simulink model "D53_LKAS"  (R2018b)
settings: Solver=ode3  StartTime=0.0  StopTime=10.0  FixedStep=0.01  RelTol=1e-3  EnableMultiTasking=on
model workspace (MAT data in the model file):
  MCOS : class17 (value not decoded)
  MCOS : class17 (value not decoded)
  MCOS : class17 (value not decoded)
  MCOS : class17 (value not decoded)
  MCOS : class17 (value not decoded)
  MCOS : class17 (value not decoded)
  MCOS : class17 (value not decoded)
  MCOS : class17 (value not decoded)
  MCOS : class17 (value not decoded)
  MCOS : class17 (value not decoded)
  MCOS : class17 (value not decoded)
  MCOS : class17 (value not decoded)
  MCOS : class17 (value not decoded)
  MCOS : class17 (value not decoded)
  MCOS : class17 (value not decoded)
  MCOS : class17 (value not decoded)
  MCOS : class17 (value not decoded)
  MCOS : class17 (value not decoded)
  MCOS : class17 (value not decoded)
  MCOS : class17 (value not decoded)
  MCOS : class17 (value not decoded)
  MCOS : class17 (value not decoded)
  MCOS : class17 (value not decoded)
  MCOS : class17 (value not decoded)
  MCOS : class17 (value not decoded)
  MCOS : class17 (value not decoded)
  MCOS : class17 (value not decoded)
  MCOS : class17 (value not decoded)
  MCOS : class17 (value not decoded)
  MCOS : class17 (value not decoded)
  MCOS : class17 (value not decoded)
  MCOS : class17 (value not decoded)
  MCOS : class17 (value not decoded)
  MCOS : class17 (value not decoded)
  MCOS : class17 (value not decoded)
  MCOS : class17 (value not decoded)
  MCOS : class17 (value not decoded)
  MCOS : class17 (value not decoded)
  MCOS : class17 (value not decoded)
  MCOS : class17 (value not decoded)
  MCOS : class17 (value not decoded)
  MCOS : class17 (value not decoded)
  MCOS : class17 (value not decoded)
  MCOS : class17 (value not decoded)
  MCOS : class17 (value not decoded)
  MCOS : class17 (value not decoded)
  MCOS : class17 (value not decoded)
  MCOS : class17 (value not decoded)
  MCOS : class17 (value not decoded)
  MCOS : class17 (value not decoded)
  MCOS : class17 (value not decoded)
  MCOS : class17 (value not decoded)
  MCOS : class17 (value not decoded)
  MCOS : class17 (value not decoded)
  MCOS : class17 (value not decoded)
  MCOS : class17 (value not decoded)
  MCOS : class17 (value not decoded)
  MCOS : class17 (value not decoded)
  MCOS : class17 (value not decoded)
  MCOS : class17 (value not decoded)
  MCOS : class17 (value not decoded)
  MCOS : class17 (value not decoded)
  MCOS : class17 (value not decoded)
  MCOS : class17 (value not decoded)
  MCOS : class17 (value not decoded)
  MCOS : class17 (value not decoded)
  MCOS : class17 (value not decoded)
  MCOS : class17 (value not decoded)
  MCOS : class17 (value not decoded)
  MCOS : class17 (value not decoded)
  MCOS : class17 (value not decoded)
  MCOS : class17 (value not decoded)
  MCOS : class17 (value not decoded)
  MCOS : class17 (value not decoded)
  MCOS : class17 (value not decoded)
  MCOS : class17 (value not decoded)
  MCOS : class17 (value not decoded)
  MCOS : class17 (value not decoded)
  MCOS : class17 (value not decoded)
  MCOS : class17 (value not decoded)
  MCOS : class17 (value not decoded)
  MCOS : class17 (value not decoded)
  MCOS : class17 (value not decoded)
  MCOS : class17 (value not decoded)
  MCOS : class17 (value not decoded)
  MCOS : class17 (value not decoded)
  MCOS : class17 (value not decoded)
  MCOS : class17 (value not decoded)
  MCOS : class17 (value not decoded)
values from neighbouring files (symbols this model uses):
  C = who    [Data_Made_Data.m]    (also in Data_Make_Data.m; Data_Process.m)
  LKA_SampleTime = Simulink.Parameter    [Model_NoProtect_Script.m]
  Monitor = find_system(strcat(filename,'/CAN Monitor (CANMon)/Monitor'),'SearchDepth',1,'BlockType','From')    [UpdateMon.m]    (also in UpdateMonAuto.m = find_system(strcat(scriptfile,'/CAN Monitor (CANMon)/Monitor; UpdateMonMdb.m; Update_MonAuto.m = find_system(strcat(scriptfile,'/CAN Monitor (CANMon)/Monitor; Update_MonMdb.m)
undefined symbols (not defined in the file or in its folder): LKA_CarWidth, LKA_StrRatio_C, LKA_Veh2CamL_C, LKA_Veh2CamW_C, LKA_WhlBaseL_C, LL_CompSWA_C, LL_CrvtPrvwT_C, LL_DesDvt_C, LL_DvtComp_C, LL_DvtPrvwT_C, LL_DvtSpdDet_vDvtSpdMin_C, LL_HdAgExT_C, LL_HdAgPrvwT_C, LL_LAccMax_C, LL_LAccRMax_C, LL_LDW_EarliestWarnLine_C, LL_LDW_LatestWarnLine_C, LL_LDWS_SUPPRESS_HEADING, LL_LFClb_TFC_DiffCtlBalance, LL_LFClb_TFC_DiffCtrlMaxSWA, LL_LFClb_TFC_DiffCtrlRatio, LL_LFClb_TFC_facmGainLutGain1_C, LL_LFClb_TFC_facmGainLutGain2_C, LL_LFClb_TFC_facmIntegRatio, LL_LFClb_TFC_facmKlat_C, LL_LFClb_TFC_FfCtlRatio_C, LL_LFClb_TFC_phiIntegCtlMaxSWA_C, LL_LFClb_TFC_tiKlatPrvwT_C, LL_LFClb_TFC_vGainLutVehSpdLwr_C, LL_LFClb_TFC_vGainLutVehSpdUpr_C, LL_LKA_EarliestWarnLine_C, LL_LKA_LatestWarnLine_C, LL_LKAExPrcs_ExitC0Dvt, LL_LKAExPrcs_ExitC0Swt, LL_LKAExPrcs_tiExitTime1, LL_LKAExPrcs_tiExitTime2, LL_LKAExPrcs_tiExitTime3, LL_LKAS_OUT_OF_CONTROL_LAT_VEL, LL_LKAS_OUT_OF_CONTROL_TTLC, LL_LKASWASyn_M0, LL_LKASWASyn_M1, LL_LKASWASyn_M2, LL_LKASWASyn_M3K, LL_LKASWASyn_SWAaddMax, LL_LKASWASyn_T2, LL_LKASWASyn_tiTrqSwaRtTime, LL_LKASWASyn_tiTrqSwaTime, LL_LKASWASyn_TrqMax, LL_LKASWASyn_TrqSwaAddSwt, LL_LKASWASyn_TrqSwaRateDiff, LL_LSpdCompT_C, LL_lStpLngth_C, LL_MAX_DELAY_EPSSTAR_TIME, LL_MAX_DRIVER_TORQUE_DISABLE, LL_MAX_DRIVER_TORQUE_ENABLE, LL_MAX_LANE_WIDTH_DISABLE, LL_MAX_LANE_WIDTH_ENABLE, LL_MAX_LAT_ACC_DISABLE, LL_MAX_LAT_ACC_ENABLE, LL_MAX_LDWS_SPEED_DISABLE ... (+29)
libraries: simulink x134, canmsglib x36, dspstat3 x3, simulink_extras x1
(part 6 of 17)

== system D53_LKAS/SignalBusCreator/bsVehMovInfo ==
  Bus Creator9 : BusCreator  Inputs=10
  CAN Recv (CANRx]) : S-Function  FunctionName=CAN_Rec_P  Parameters=uint8(Module-1),uint32(ID),uint8(Frameformat-1),uint8(Newflag),uint8(FIFO),double(sampletime)  SFunctionDeploymentMode=off  EnableBusSupport=off  mask(CAN_receive){Module=CAN_1, ID=973, Frameformat=Standard (11-bit identifier), Newflag=off, FIFO=off, sampletime=0.01}
      mask prompts: Module "CAN Port:"; ID "CAN Frame ID:"; Frameformat "CAN Frame Format:"; FIFO "Overflow flag"
      mask init:
      | maskdisplay = canrecicon(Module,ID,Frameformat,Newflag,FIFO);
      | set_param(gcb, 'MaskDisplay', maskdisplay);
      mask TypeOptions Module: CAN_0 | CAN_1 | CAN_2 | CAN_3
      mask TypeOptions Frameformat: Standard (11-bit identifier) | Extended (29-bit identifier)
      mask Display: color('blue');text(0.98,0.9,'MPC5675K','horizontalAlignment','right');color('black');text(0.5,0.6,'FlexCAN_1 Receive','horizontalAlignment','center');text(0.5,0.35,'Standard ID:973','horizontalAlignment','center');port_label('output',1,'CAN_Msg');
  CAN Recv (CANRx])1 : S-Function  FunctionName=CAN_Rec_P  Parameters=uint8(Module-1),uint32(ID),uint8(Frameformat-1),uint8(Newflag),uint8(FIFO),double(sampletime)  SFunctionDeploymentMode=off  EnableBusSupport=off  mask(CAN_receive){Module=CAN_1, ID=909, Frameformat=Extended (29-bit identifier), Newflag=off, FIFO=off, sampletime=0.01}
      mask prompts: Module "CAN Port:"; ID "CAN Frame ID:"; Frameformat "CAN Frame Format:"; FIFO "Overflow flag"
      mask init:
      | maskdisplay = canrecicon(Module,ID,Frameformat,Newflag,FIFO);
      | set_param(gcb, 'MaskDisplay', maskdisplay);
      mask TypeOptions Module: CAN_0 | CAN_1 | CAN_2 | CAN_3
      mask TypeOptions Frameformat: Standard (11-bit identifier) | Extended (29-bit identifier)
      mask Display: color('blue');text(0.98,0.9,'MPC5675K','horizontalAlignment','right');color('black');text(0.5,0.6,'FlexCAN_1 Receive','horizontalAlignment','center');text(0.5,0.35,'Extended ID:909','horizontalAlignment','center');port_label('output',1,'CAN_Msg');
  CAN Send1 : S-Function  FunctionName=CAN_Send_P  Parameters=uint8(CAN_Port-1),uint8(CAN_Priority-1),uint8(S_overflow_flag),uint8(S_timestamp),double(sampletime)  SFunctionDeploymentMode=off  EnableBusSupport=off  mask{CAN_Port=CAN_0, CAN_Priority=3, S_overflow_flag=off, S_timestamp=off, sampletime=0.01}
      mask prompts: CAN_Port "CAN Port:"; CAN_Priority "Priority:"; S_overflow_flag "Send overflow flag"; S_timestamp "Send time stamp"
      mask init:
      | maskdisplay = cansendicon(CAN_Port,CAN_Priority,S_overflow_flag,S_timestamp);
      | set_param(gcb, 'MaskDisplay', maskdisplay);
      mask TypeOptions CAN_Port: CAN_0 | CAN_1 | CAN_2 | CAN_3
      mask TypeOptions CAN_Priority: 0 | 1 | 2 | 3 | 4 | 5 | 6 | 7
      mask Display: color('blue');text(0.98,0.9,'MPC5675K','horizontalAlignment','right');color('black');text(0.5,0.6,'FlexCAN_0 Send','horizontalAlignment','center');text(0.5,0.35,'Priority:3','horizontalAlignment','center');port_label('input',1,'CAN_Msg');
  CAN Send2 : S-Function  FunctionName=CAN_Send_P  Parameters=uint8(CAN_Port-1),uint8(CAN_Priority-1),uint8(S_overflow_flag),uint8(S_timestamp),double(sampletime)  SFunctionDeploymentMode=off  EnableBusSupport=off  mask{CAN_Port=CAN_0, CAN_Priority=3, S_overflow_flag=off, S_timestamp=off, sampletime=0.01}
      mask prompts: CAN_Port "CAN Port:"; CAN_Priority "Priority:"; S_overflow_flag "Send overflow flag"; S_timestamp "Send time stamp"
      mask init:
      | maskdisplay = cansendicon(CAN_Port,CAN_Priority,S_overflow_flag,S_timestamp);
      | set_param(gcb, 'MaskDisplay', maskdisplay);
      mask TypeOptions CAN_Port: CAN_0 | CAN_1 | CAN_2 | CAN_3
      mask TypeOptions CAN_Priority: 0 | 1 | 2 | 3 | 4 | 5 | 6 | 7
      mask Display: color('blue');text(0.98,0.9,'MPC5675K','horizontalAlignment','right');color('black');text(0.5,0.6,'FlexCAN_0 Send','horizontalAlignment','center');text(0.5,0.35,'Priority:3','horizontalAlignment','center');port_label('input',1,'CAN_Msg');
  CAN Send3 : S-Function  FunctionName=CAN_Send_P  Parameters=uint8(CAN_Port-1),uint8(CAN_Priority-1),uint8(S_overflow_flag),uint8(S_timestamp),double(sampletime)  SFunctionDeploymentMode=off  EnableBusSupport=off  mask{CAN_Port=CAN_0, CAN_Priority=3, S_overflow_flag=off, S_timestamp=off, sampletime=0.01}
      mask prompts: CAN_Port "CAN Port:"; CAN_Priority "Priority:"; S_overflow_flag "Send overflow flag"; S_timestamp "Send time stamp"
      mask init:
      | maskdisplay = cansendicon(CAN_Port,CAN_Priority,S_overflow_flag,S_timestamp);
      | set_param(gcb, 'MaskDisplay', maskdisplay);
      mask TypeOptions CAN_Port: CAN_0 | CAN_1 | CAN_2 | CAN_3
      mask TypeOptions CAN_Priority: 0 | 1 | 2 | 3 | 4 | 5 | 6 | 7
      mask Display: color('blue');text(0.98,0.9,'MPC5675K','horizontalAlignment','right');color('black');text(0.5,0.6,'FlexCAN_0 Send','horizontalAlignment','center');text(0.5,0.35,'Priority:3','horizontalAlignment','center');port_label('input',1,'CAN_Msg');
  CAN Unpack : canmsglib/CAN Unpack  CANdbFile=D:\Work\02_LKA\LKAS\Documents\D53-PSA1CAN.dbc  MsgList=ESC_3CD_PSA1  MsgName=ESC_3CD_PSA1  MsgIDType=Standard (11-bit identifier)  MsgIdentifier=973  MsgLength=8  SignalInfo=Brake_pedal_disabled_UC_Brake$37$1$2$2$1$0$1$0$-Inf$Inf$#Frame_checksum3CD$60$4$2$2$1$0$1$0$-Inf$Inf$#Lateral_acceleration$8$16$2$1$1$0$5.000000e-02$0$-15$15$#TMC_pressure$52$12$2$2$1$0$1.000000e-01$-55$-55$3.544000e+02$#Yaw_speed$24$16$2$1$1$0$1.000000e-01$0$-100$100$#bits_compute_process_counter3CD$56$4$2$2$1$0$1$0$0$15$#  NSignals=6  IDPort=off  TimestampPort=off  ErrorPort=off  RemotePort=off  LengthPort=off  StatusPort=off  StartBits=str2num('[int32(37);int32(60);int32(8);int32(52);int32(24);int32(56)]')  SignalSizes=str2num('[int32(1);int32(4);int32(16);int32(12);int32(16);int32(4)]')  ByteOrders=str2num('[int32(2);int32(2);int32(2);int32(2);int32(2);int32(2)]')  DataTypes=str2num('[int32(2);int32(2);int32(1);int32(2);int32(1);int32(2)]')  MultiplexTypes=str2num('[int32(1);int32(1);int32(1);int32(1);int32(1);int32(1)]')  MultiplexValues=str2num('[double(0);double(0);double(0);double(0);double(0);double(0)]')  Factors=str2num('[double(1);double(1);double(5.000000e-02);double(1.000000e-01);double(1.000000e-01);double(1)]')  Offsets=str2num('[double(0);double(0);double(0);double(-55);double(0);double(0)]')  Minimums=str2num('[double(-Inf);double(-Inf);double(-15);double(-55);double(-100);double(0)]')  Maximums=str2num('[double(Inf);double(Inf);double(15);double(3.544000e+02);double(100);double(15)]')  ApplyMinMax=off
      settings: SourceProductName=Simulink Real-Time  SourceProductBaseCode=XP  DataFormat=CANdb specified signals
  CAN Unpack1 : canmsglib/CAN Unpack  CANdbFile=D:\Work\02_LKA\LKAS\Documents\D53-PSA1CAN.dbc  MsgList=ESC_38D_PSA1  MsgName=ESC_38D_PSA1  MsgIDType=Standard (11-bit identifier)  MsgIdentifier=909  MsgLength=8  SignalInfo=ABR_dynamic_checksum$40$4$2$2$1$0$1$0$-Inf$Inf$#Vehicle_driving_direction$52$2$2$2$1$0$1$0$-Inf$Inf$#Vehicle_speed_of_wheelsensor$8$16$2$2$1$0$1.000000e-02$0$0$6.553400e+02$#Vehiclespeed_unavailability_flag$50$2$2$2$1$0$1$0$-Inf$Inf$#bits_compute_for_UC_brake$44$4$2$2$1$0$1$0$0$15$#  NSignals=5  IDPort=off  TimestampPort=off  ErrorPort=off  RemotePort=off  LengthPort=off  StatusPort=off  StartBits=str2num('[int32(40);int32(52);int32(8);int32(50);int32(44)]')  SignalSizes=str2num('[int32(4);int32(2);int32(16);int32(2);int32(4)]')  ByteOrders=str2num('[int32(2);int32(2);int32(2);int32(2);int32(2)]')  DataTypes=str2num('[int32(2);int32(2);int32(2);int32(2);int32(2)]')  MultiplexTypes=str2num('[int32(1);int32(1);int32(1);int32(1);int32(1)]')  MultiplexValues=str2num('[double(0);double(0);double(0);double(0);double(0)]')  Factors=str2num('[double(1);double(1);double(1.000000e-02);double(1);double(1)]')  Offsets=str2num('[double(0);double(0);double(0);double(0);double(0)]')  Minimums=str2num('[double(-Inf);double(-Inf);double(0);double(-Inf);double(0)]')  Maximums=str2num('[double(Inf);double(Inf);double(6.553400e+02);double(Inf);double(15)]')  ApplyMinMax=off
      settings: SourceProductName=Simulink Real-Time  SourceProductBaseCode=XP  DataFormat=CANdb specified signals
  CAN Unpack4 : canmsglib/CAN Unpack  CANdbFile=D:\Work\02_LKA\LKAS\Documents\D53-PSA1CAN.dbc  MsgList=GW_32D_PSA1  MsgName=GW_32D_PSA1  MsgIDType=Standard (11-bit identifier)  MsgIdentifier=813  MsgLength=8  SignalInfo=ACCEL_LONGI_CALIB$12$12$2$2$1$0$2.000000e-02$-4.096000e+01$-4.096000e+01$4.092000e+01$#Brake_Pedal_Active$16$2$2$2$1$0$1$0$-Inf$Inf$#Braking_effort$9$1$2$2$1$0$1$0$-Inf$Inf$#ESC_ACC_Status$19$2$2$2$1$0$1$0$-Inf$Inf$#ESC_AEB_Status$10$2$2$2$1$0$1$0$-Inf$Inf$#Message_from_ESC_informing$23$1$2$2$1$0$1$0$-Inf$Inf$#UFC_to_ACC_dynamic_frame$56$4$2$2$1$0$1$0$-Inf$Inf$#Vehicle_Hold_Status$29$2$2$2$1$0$1$0$-Inf$Inf$#Vehicle_detected_as_stationary$21$1$2$2$1$0$1$0$-Inf$Inf$#YawRate_Raw$44$12$2$2$1$0$8.000000e-02$-1.638400e+02$-1.638400e+02$1.636800e+02$#bits_compute_counter_for_UCbrake$60$4$2$2$1$0$1$0$0$15$#  NSignals=11  IDPort=off  TimestampPort=off  ErrorPort=off  RemotePort=off  LengthPort=off  StatusPort=off  StartBits=str2num('[int32(12);int32(16);int32(9);int32(19);int32(10);int32(23);int32(56);int32(29);int32(21);int32(44);int32(60)]')  SignalSizes=str2num('[int32(12);int32(2);int32(1);int32(2);int32(2);int32(1);int32(4);int32(2);int32(1);int32(12);int32(4)]')  ByteOrders=str2num('[int32(2);int32(2);int32(2);int32(2);int32(2);int32(2);int32(2);int32(2);int32(2);int32(2);int32(2)]')  DataTypes=str2num('[int32(2);int32(2);int32(2);int32(2);int32(2);int32(2);int32(2);int32(2);int32(2);int32(2);int32(2)]')  MultiplexTypes=str2num('[int32(1);int32(1);int32(1);int32(1);int32(1);int32(1);int32(1);int32(1);int32(1);int32(1);int32(1)]')  MultiplexValues=str2num('[double(0);double(0);double(0);double(0);double(0);double(0);double(0);double(0);double(0);double(0);double(0)]')  Factors=str2num('[double(2.000000e-02);double(1);double(1);double(1);double(1);double(1);double(1);double(1);double(1);double(8.000000e-02);double(1)]')  Offsets=str2num('[double(-4.096000e+01);double(0);double(0);double(0);double(0);double(0);double(0);double(0);double(0);double(-1.638400e+02);double(0)]')  Minimums=str2num('[double(-4.096000e+01);double(-Inf);double(-Inf);double(-Inf);double(-Inf);double(-Inf);double(-Inf);double(-Inf);double(-Inf);double(-1.638400e+02);double(0)]')  Maximums=str2num('[double(4.092000e+01);double(Inf);double(Inf);double(Inf);double(Inf);double(Inf);double(Inf);double(Inf);double(Inf);double(1.636800e+02);double(15)]')  ApplyMinMax=off
      settings: SourceProductName=Simulink Real-Time  SourceProductBaseCode=XP  DataFormat=CANdb specified signals
  CAN_Receive4 : S-Function  FunctionName=CAN_Rec_P  Parameters=uint8(Module-1),uint32(ID),uint8(Frameformat-1),uint8(Newflag),uint8(FIFO),double(sampletime)  SFunctionDeploymentMode=off  EnableBusSupport=off  mask(CAN_receive){Module=CAN_1, ID=813, Frameformat=Standard (11-bit identifier), Newflag=off, FIFO=off, sampletime=0.01}
      mask prompts: Module "CAN Port:"; ID "CAN Frame ID:"; Frameformat "CAN Frame Format:"; FIFO "Overflow flag"
      mask init:
      | maskdisplay = canrecicon(Module,ID,Frameformat,Newflag,FIFO);
      | set_param(gcb, 'MaskDisplay', maskdisplay);
      mask TypeOptions Module: CAN_0 | CAN_1 | CAN_2 | CAN_3
      mask TypeOptions Frameformat: Standard (11-bit identifier) | Extended (29-bit identifier)
      mask Display: color('blue');text(0.98,0.9,'MPC5675K','horizontalAlignment','right');color('black');text(0.5,0.6,'FlexCAN_1 Receive','horizontalAlignment','center');text(0.5,0.35,'Standard ID:813','horizontalAlignment','center');port_label('output',1,'CAN_Msg');
  Data Type Conversion{1..5,11} (6 alike) : DataTypeConversion  OutDataTypeStr=single
  Data Type Conversion53 : DataTypeConversion  OutDataTypeStr=uint8
  Ground : Ground
  Ground1 : Ground
  Ground2 : Ground
  Rate Transition{,1..5,7} (7 alike) : RateTransition  OutPortSampleTime=0.01
  Terminator{,1..14} (15 alike) : Terminator
  bsVehMovInfo : Outport
  wires:
  CAN Unpack4/1 -> Rate Transition/1
  CAN Unpack/3 -> Rate Transition3/1
  CAN Unpack1/4 -> Rate Transition4/1
  Data Type Conversion2/1 -> Bus Creator9/3  "ESC_YawRate"
  Ground1/1 -> Bus Creator9/4  "ESC_YawRate_Valid"
  Rate Transition3/1 -> Data Type Conversion3/1
  CAN Unpack4/6 -> Terminator7/1
  CAN Unpack/1 -> Terminator2/1
  Rate Transition2/1 -> Data Type Conversion2/1
  Rate Transition7/1 -> Data Type Conversion5/1
  CAN Recv (CANRx])/1 -> CAN Send2/1, CAN Unpack/1
  CAN Unpack1/3 -> Rate Transition7/1
  Data Type Conversion4/1 -> Bus Creator9/5  "ESC_UnYawRate"
  Data Type Conversion11/1 -> Bus Creator9/7  "ESC_LonAcc"
  CAN Unpack/4 -> Rate Transition1/1
  Data Type Conversion53/1 -> Bus Creator9/10  "ESC_VehSpd_Valid"
  Data Type Conversion3/1 -> Bus Creator9/1  "ESC_LatAcc"
  Rate Transition4/1 -> Data Type Conversion53/1
  Rate Transition5/1 -> Data Type Conversion4/1
  Ground2/1 -> Bus Creator9/2  "ESC_LatAcc_Valid"
  Rate Transition1/1 -> Data Type Conversion1/1
  CAN Unpack4/10 -> Rate Transition5/1
  Data Type Conversion1/1 -> Bus Creator9/9  "ESC_Brake_Press"
  CAN Unpack/5 -> Rate Transition2/1
  Rate Transition/1 -> Data Type Conversion11/1
  CAN Unpack4/11 -> Terminator11/1
  CAN Unpack/6 -> Terminator1/1
  Data Type Conversion5/1 -> Bus Creator9/6  "ESC_VehSpd"
  CAN Unpack/2 -> Terminator/1
  CAN Unpack4/4 -> Terminator5/1
  CAN_Receive4/1 -> CAN Send1/1, CAN Unpack4/1
  CAN Unpack4/8 -> Terminator9/1
  CAN Unpack4/7 -> Terminator8/1
  CAN Unpack4/5 -> Terminator6/1
  CAN Unpack4/9 -> Terminator10/1
  CAN Unpack4/2 -> Terminator3/1
  CAN Unpack4/3 -> Terminator4/1
  Bus Creator9/1 -> bsVehMovInfo/1  "bsVehMovInfo"
  Ground/1 -> Bus Creator9/8  "ESC_LonAcc_Valid"
  CAN Recv (CANRx])1/1 -> CAN Send3/1, CAN Unpack1/1
  CAN Unpack1/1 -> Terminator12/1
  CAN Unpack1/2 -> Terminator13/1
  CAN Unpack1/5 -> Terminator14/1

== system D53_LKAS/Clb/Calibration1/Subsystem2 ==
  In1 : Inport
  In2 : Inport  Port=2
  In3 : Inport  Port=3
  In4 : Inport  Port=4
  In5 : Inport  Port=5
  In6 : Inport  Port=6
  In7 : Inport  Port=7
  In8 : Inport  Port=8
  In9 : Inport  Port=9
  In10 : Inport  Port=10
  In11 : Inport  Port=11
  If Action Subsystem : Subsystem  TreatAsAtomicUnit=on
  If Action Subsystem1 : Subsystem  TreatAsAtomicUnit=on
  If Action Subsystem2 : Subsystem  TreatAsAtomicUnit=on
  If Action Subsystem3 : Subsystem  TreatAsAtomicUnit=on
  If Action Subsystem4 : Subsystem  TreatAsAtomicUnit=on
  If Action Subsystem5 : Subsystem  TreatAsAtomicUnit=on
  If Action Subsystem6 : Subsystem  TreatAsAtomicUnit=on
  If Action Subsystem7 : Subsystem  TreatAsAtomicUnit=on
  If Action Subsystem8 : Subsystem  TreatAsAtomicUnit=on
  If Action Subsystem9 : Subsystem  TreatAsAtomicUnit=on
  Out1 : Outport
  Out2 : Outport  Port=2
  Out3 : Outport  Port=3
  Out4 : Outport  Port=4
  Out5 : Outport  Port=5
  Out6 : Outport  Port=6
  Out7 : Outport  Port=7
  Out8 : Outport  Port=8
  Out9 : Outport  Port=9
  Out10 : Outport  Port=10
  wires:
  If Action Subsystem8/1(Out1) -> Out9/1
  In9/1 -> If Action Subsystem8/Action
  If Action Subsystem7/1(Out1) -> Out8/1
  In8/1 -> If Action Subsystem7/Action
  If Action Subsystem6/1(Out1) -> Out7/1
  In7/1 -> If Action Subsystem6/Action
  If Action Subsystem5/1(Out1) -> Out6/1
  In6/1 -> If Action Subsystem5/Action
  If Action Subsystem4/1(Out1) -> Out5/1
  In5/1 -> If Action Subsystem4/Action
  If Action Subsystem3/1(Out1) -> Out4/1
  In4/1 -> If Action Subsystem3/Action
  If Action Subsystem2/1(Out1) -> Out3/1
  In3/1 -> If Action Subsystem2/Action
  If Action Subsystem1/1(Out1) -> Out2/1
  In2/1 -> If Action Subsystem1/Action
  If Action Subsystem/1(Out1) -> Out1/1
  In1/1 -> If Action Subsystem/Action
  If Action Subsystem9/1(Out1) -> Out10/1
  In10/1 -> If Action Subsystem9/Action
  In11/1 -> If Action Subsystem/1(In1), If Action Subsystem1/1(In1), If Action Subsystem2/1(In1), If Action Subsystem3/1(In1), If Action Subsystem4/1(In1), If Action Subsystem5/1(In1), If Action Subsystem6/1(In1), If Action Subsystem7/1(In1), If Action Subsystem8/1(In1), If Action Subsystem9/1(In1)

== system D53_LKAS/Clb/Calibration2/Subsystem2 ==
  In1 : Inport
  In2 : Inport  Port=2
  In3 : Inport  Port=3
  In4 : Inport  Port=4
  In5 : Inport  Port=5
  In6 : Inport  Port=6
  In7 : Inport  Port=7
  In8 : Inport  Port=8
  In9 : Inport  Port=9
  In10 : Inport  Port=10
  In11 : Inport  Port=11
  If Action Subsystem : Subsystem  TreatAsAtomicUnit=on
  If Action Subsystem1 : Subsystem  TreatAsAtomicUnit=on
  If Action Subsystem2 : Subsystem  TreatAsAtomicUnit=on
  If Action Subsystem3 : Subsystem  TreatAsAtomicUnit=on
  If Action Subsystem4 : Subsystem  TreatAsAtomicUnit=on
  If Action Subsystem5 : Subsystem  TreatAsAtomicUnit=on
  If Action Subsystem6 : Subsystem  TreatAsAtomicUnit=on
  If Action Subsystem7 : Subsystem  TreatAsAtomicUnit=on
  If Action Subsystem8 : Subsystem  TreatAsAtomicUnit=on
  If Action Subsystem9 : Subsystem  TreatAsAtomicUnit=on
  Out1 : Outport
  Out2 : Outport  Port=2
  Out3 : Outport  Port=3
  Out4 : Outport  Port=4
  Out5 : Outport  Port=5
  Out6 : Outport  Port=6
  Out7 : Outport  Port=7
  Out8 : Outport  Port=8
  Out9 : Outport  Port=9
  Out10 : Outport  Port=10
  wires:
  In11/1 -> If Action Subsystem9/1(In1), If Action Subsystem8/1(In1), If Action Subsystem7/1(In1), If Action Subsystem6/1(In1), If Action Subsystem5/1(In1), If Action Subsystem4/1(In1), If Action Subsystem3/1(In1), If Action Subsystem2/1(In1), If Action Subsystem1/1(In1), If Action Subsystem/1(In1)
  In10/1 -> If Action Subsystem9/Action
  If Action Subsystem9/1(Out1) -> Out10/1
  In1/1 -> If Action Subsystem/Action
  If Action Subsystem/1(Out1) -> Out1/1
  In2/1 -> If Action Subsystem1/Action
  If Action Subsystem1/1(Out1) -> Out2/1
  In3/1 -> If Action Subsystem2/Action
  If Action Subsystem2/1(Out1) -> Out3/1
  In4/1 -> If Action Subsystem3/Action
  If Action Subsystem3/1(Out1) -> Out4/1
  In5/1 -> If Action Subsystem4/Action
  If Action Subsystem4/1(Out1) -> Out5/1
  In6/1 -> If Action Subsystem5/Action
  If Action Subsystem5/1(Out1) -> Out6/1
  In7/1 -> If Action Subsystem6/Action
  If Action Subsystem6/1(Out1) -> Out7/1
  In8/1 -> If Action Subsystem7/Action
  If Action Subsystem7/1(Out1) -> Out8/1
  In9/1 -> If Action Subsystem8/Action
  If Action Subsystem8/1(Out1) -> Out9/1

== system D53_LKAS/Clb/Calibration3/Subsystem2 ==
  In1 : Inport
  In2 : Inport  Port=2
  In3 : Inport  Port=3
  In4 : Inport  Port=4
  In5 : Inport  Port=5
  In6 : Inport  Port=6
  In7 : Inport  Port=7
  In8 : Inport  Port=8
  In9 : Inport  Port=9
  In10 : Inport  Port=10
  In11 : Inport  Port=11
  If Action Subsystem : Subsystem  TreatAsAtomicUnit=on
  If Action Subsystem1 : Subsystem  TreatAsAtomicUnit=on
  If Action Subsystem2 : Subsystem  TreatAsAtomicUnit=on
  If Action Subsystem3 : Subsystem  TreatAsAtomicUnit=on
  If Action Subsystem4 : Subsystem  TreatAsAtomicUnit=on
  If Action Subsystem5 : Subsystem  TreatAsAtomicUnit=on
  If Action Subsystem6 : Subsystem  TreatAsAtomicUnit=on
  If Action Subsystem7 : Subsystem  TreatAsAtomicUnit=on
  If Action Subsystem8 : Subsystem  TreatAsAtomicUnit=on
  If Action Subsystem9 : Subsystem  TreatAsAtomicUnit=on
  Out1 : Outport
  Out2 : Outport  Port=2
  Out3 : Outport  Port=3
  Out4 : Outport  Port=4
  Out5 : Outport  Port=5
  Out6 : Outport  Port=6
  Out7 : Outport  Port=7
  Out8 : Outport  Port=8
  Out9 : Outport  Port=9
  Out10 : Outport  Port=10
  wires:
  If Action Subsystem8/1(Out1) -> Out9/1
  In9/1 -> If Action Subsystem8/Action
  If Action Subsystem7/1(Out1) -> Out8/1
  In8/1 -> If Action Subsystem7/Action
  If Action Subsystem6/1(Out1) -> Out7/1
  In7/1 -> If Action Subsystem6/Action
  If Action Subsystem5/1(Out1) -> Out6/1
  In6/1 -> If Action Subsystem5/Action
  If Action Subsystem4/1(Out1) -> Out5/1
  In5/1 -> If Action Subsystem4/Action
  If Action Subsystem3/1(Out1) -> Out4/1
  In4/1 -> If Action Subsystem3/Action
  If Action Subsystem2/1(Out1) -> Out3/1
  In3/1 -> If Action Subsystem2/Action
  If Action Subsystem1/1(Out1) -> Out2/1
  In2/1 -> If Action Subsystem1/Action
  If Action Subsystem/1(Out1) -> Out1/1
  In1/1 -> If Action Subsystem/Action
  If Action Subsystem9/1(Out1) -> Out10/1
  In10/1 -> If Action Subsystem9/Action
  In11/1 -> If Action Subsystem/1(In1), If Action Subsystem1/1(In1), If Action Subsystem2/1(In1), If Action Subsystem3/1(In1), If Action Subsystem4/1(In1), If Action Subsystem5/1(In1), If Action Subsystem6/1(In1), If Action Subsystem7/1(In1), If Action Subsystem8/1(In1), If Action Subsystem9/1(In1)

== system D53_LKAS/LL/Human Machine Interface (HMI)/Subsystem ==
  LDW_STATE : Inport
  EPSInfo : Inport  Port=2
  Abs : Abs
  Bus Selector2 : BusSelector  OutputSignals=EPS_LKA_State,EPS_SW_Trq
  Compare1 : simulink/Logic and Bit Operations/Compare To Constant  relop===  const=3  OutDataTypeStr=boolean
  Compare2 : simulink/Logic and Bit Operations/Compare To Constant  relop===  const=3  OutDataTypeStr=boolean
  Compare3 : simulink/Logic and Bit Operations/Compare To Constant  relop===  const=1  OutDataTypeStr=boolean
  Compare4 : simulink/Logic and Bit Operations/Compare To Constant  relop===  const=3  OutDataTypeStr=boolean
  Compare5 : simulink/Logic and Bit Operations/Compare To Constant  relop===  const=4  OutDataTypeStr=boolean
  Compare6 : simulink/Logic and Bit Operations/Compare To Constant  relop===  const=5  OutDataTypeStr=boolean
  Constant : Constant  Value=0.25  OutDataTypeStr=single
  Constant1 : Constant  Value=0.5  OutDataTypeStr=single
  Count 10s : Subsystem
  Count 15s : Subsystem
  Logical Operator2 : Logic  AllPortsSameDT=off  OutDataTypeStr=boolean
  Logical Operator3 : Logic  Operator=OR  Inputs=5  AllPortsSameDT=off  OutDataTypeStr=boolean
  Relational Operator : RelationalOperator  Operator=<=  OutDataTypeStr=boolean  RndMeth=Nearest
  Switch : Switch  Criteria=u2 > Threshold
  HandsOff10s : Outport
  HandsOff15s : Outport  Port=2
  wires:
  Abs/1 -> Relational Operator/1
  Compare6/1 -> Logical Operator3/1
  Compare5/1 -> Logical Operator3/2
  Compare4/1 -> Logical Operator3/3
  LDW_STATE/1 -> Compare5/1, Compare6/1, Compare4/1
  Count 15s/1(Out) -> HandsOff15s/1
  Relational Operator/1 -> Logical Operator2/2
  Constant1/1 -> Switch/1
  Logical Operator3/1 -> Logical Operator2/1
  Logical Operator2/1 -> Count 10s/Enable, Count 15s/Enable
  Bus Selector2/2 -> Abs/1  "<EPS_SW_Trq>"
  Compare1/1 -> Switch/2
  Switch/1 -> Relational Operator/2
  EPSInfo/1 -> Bus Selector2/1
  Constant/1 -> Switch/3
  Bus Selector2/1 -> Compare2/1, Compare3/1, Compare1/1  "<EPS_LKA_State>"
  Compare2/1 -> Logical Operator3/4
  Compare3/1 -> Logical Operator3/5
  Count 10s/1(Out) -> HandsOff10s/1

== system D53_LKAS/LL/LL Inputs Mapping/bsBCMInfo ==
  bsBCMInfoIn : Inport
  Bus Creator1 : BusCreator  Inputs=3
  Bus Selector1 : BusSelector  OutputSignals=BCM_Double_Light,BCM_Left_Light,BCM_Right_Light
  bsBCMInfoOut : Outport
  wires:
  bsBCMInfoIn/1 -> Bus Selector1/1
  Bus Selector1/1 -> Bus Creator1/1  "<BCM_Double_Light>"
  Bus Creator1/1 -> bsBCMInfoOut/1
  Bus Selector1/2 -> Bus Creator1/2  "<BCM_Left_Light>"
  Bus Selector1/3 -> Bus Creator1/3  "<BCM_Right_Light>"

== system D53_LKAS/LL/LL Inputs Mapping/bsEPSInfo ==
  bsEPSInfoIn : Inport
  Bus Creator4 : BusCreator  Inputs=9
  Bus Selector1 : BusSelector  OutputSignals=EPS_LKA_State,EPS_SW_Trq,EPS_Error_State,EPS_Trq_State,SAS_Clb_State,SAS_Trim_State,EPS_TrqLim_State,EPS_LKA_Current,EPS_SWHold_State
  bsEPSInfoOut : Outport
  wires:
  bsEPSInfoIn/1 -> Bus Selector1/1
  Bus Selector1/2 -> Bus Creator4/2  "<EPS_SW_Trq>"
  Bus Selector1/1 -> Bus Creator4/1  "<EPS_LKA_State>"
  Bus Creator4/1 -> bsEPSInfoOut/1
  Bus Selector1/3 -> Bus Creator4/3  "<EPS_Error_State>"
  Bus Selector1/4 -> Bus Creator4/4  "<EPS_Trq_State>"
  Bus Selector1/5 -> Bus Creator4/5  "<SAS_Clb_State>"
  Bus Selector1/6 -> Bus Creator4/6  "<SAS_Trim_State>"
  Bus Selector1/7 -> Bus Creator4/7  "<EPS_TrqLim_State>"
  Bus Selector1/8 -> Bus Creator4/8  "<EPS_LKA_Current>"
  Bus Selector1/9 -> Bus Creator4/9  "<EPS_SWHold_State>"

== system D53_LKAS/LL/LL Inputs Mapping/bsLaneInfo ==
  bsLaneInfoIn : Inport
  Bus Creator : BusCreator  Inputs=7
  Bus Selector1 : BusSelector  OutputSignals=bsFusLaneInfo,bsFusL0Info,bsFusR0Info,bsFusL1Info,bsFusR1Info,bsOriLaneInfo,bsOriL0Info,bsOriR0Info,bsOriL1Info,bsOriR1Info,Fusion_AdditionalInf
  LaneSelect : Subsystem
  "LanesReconstruct " : Subsystem
  bsLaneInfoOut : Outport
  wires:
  bsLaneInfoIn/1 -> Bus Selector1/1
  Bus Selector1/11 -> Bus Creator/7  "<Fusion_AdditionalInf>"
  "LanesReconstruct "/1(bsL0InfoR) -> Bus Creator/2  "bsL0Info"
  "LanesReconstruct "/2(bsR0InfoR) -> Bus Creator/3  "bsR0Info"
  "LanesReconstruct "/3(bsL1InfoR) -> Bus Creator/4  "bsL1Info"
  "LanesReconstruct "/4(bsR1InfoR) -> Bus Creator/5  "bsR1Info"
  LaneSelect/1(bsL0Info) -> "LanesReconstruct "/1(bsL0Info)
  LaneSelect/2(bsR0Info) -> "LanesReconstruct "/2(bsR0Info)
  LaneSelect/3(bsL1Info) -> "LanesReconstruct "/3(bsL1Info)
  LaneSelect/4(bsR1Info) -> "LanesReconstruct "/4(bsR1Info)
  Bus Selector1/2 -> LaneSelect/1(bsFusL0Info)  "<bsFusL0Info>"
  Bus Selector1/3 -> LaneSelect/2(bsFusR0Info)  "<bsFusR0Info>"
  Bus Selector1/4 -> LaneSelect/3(bsFusL1Info)  "<bsFusL1Info>"
  Bus Selector1/5 -> LaneSelect/4(bsFusR1Info)  "<bsFusR1Info>"
  Bus Selector1/7 -> LaneSelect/5(bsOriL0Info)  "<bsOriL0Info>"
  Bus Selector1/8 -> LaneSelect/6(bsOriR0Info)  "<bsOriR0Info>"
  Bus Selector1/9 -> LaneSelect/7(bsOriL1Info)  "<bsOriL1Info>"
  Bus Selector1/10 -> LaneSelect/8(bsOriR1Info)  "<bsOriR1Info>"
  Bus Creator/1 -> bsLaneInfoOut/1
  Bus Selector1/6 -> Bus Creator/6  "<bsOriLaneInfo>"
  Bus Selector1/1 -> Bus Creator/1  "<bsFusLaneInfo>"

== system D53_LKAS/LL/LL Inputs Mapping/bsMP5Info ==
  bsMP5InfoIn : Inport
  Bus Creator4 : BusCreator  Inputs=3
  Bus Selector1 : BusSelector  OutputSignals=LKA_Main_Switch,LKA_Mode,LDW_Warn_Mode
  bsMP5InfoOut : Outport
  wires:
  Bus Selector1/1 -> Bus Creator4/1  "<LKA_Main_Switch>"
  Bus Selector1/2 -> Bus Creator4/2  "<LKA_Mode>"
  Bus Creator4/1 -> bsMP5InfoOut/1
  bsMP5InfoIn/1 -> Bus Selector1/1
  Bus Selector1/3 -> Bus Creator4/3  "<LDW_Warn_Mode>"

== system D53_LKAS/LL/LL Inputs Mapping/bsPTState ==
  bsPTStateIn : Inport
  Bus Creator3 : BusCreator  Inputs=2
  Bus Selector1 : BusSelector  OutputSignals=AccPedal_Pos,TCU_ActualGear
  bsPTStateOut : Outport
  wires:
  Bus Selector1/2 -> Bus Creator3/2  "<TCU_ActualGear>"
  bsPTStateIn/1 -> Bus Selector1/1
  Bus Selector1/1 -> Bus Creator3/1  "<AccPedal_Pos>"
  Bus Creator3/1 -> bsPTStateOut/1

== system D53_LKAS/LL/LL Inputs Mapping/bsSWAInfo ==
  bsSWAInfoIn : Inport
  Bus Creator : BusCreator  Inputs=4
  Bus Selector1 : BusSelector  OutputSignals=SW_Angle,SW_Angle_Speed,SWS_Fault_Code,SAS_In_Status
  bsSWAInfoOut : Outport
  wires:
  bsSWAInfoIn/1 -> Bus Selector1/1
  Bus Selector1/1 -> Bus Creator/1  "<SW_Angle>"
  Bus Selector1/2 -> Bus Creator/2  "<SW_Angle_Speed>"
  Bus Selector1/3 -> Bus Creator/3  "<SWS_Fault_Code>"
  Bus Selector1/4 -> Bus Creator/4  "<SAS_In_Status>"
  Bus Creator/1 -> bsSWAInfoOut/1

== system D53_LKAS/LL/LL Inputs Mapping/bsVehMovInfo ==
  bsVehMovInfoIn : Inport
  Bus Creator : BusCreator  Inputs=10
  Bus Selector2 : BusSelector  OutputSignals=ESC_LatAcc,ESC_LatAcc_Valid,ESC_YawRate,ESC_YawRate_Valid,ESC_UnYawRate,ESC_VehSpd,ESC_LonAcc,ESC_LonAcc_Valid,ESC_Brake_Press,ESC_VehSpd_Valid
  bsVehMovInfoOut : Outport
  wires:
  bsVehMovInfoIn/1 -> Bus Selector2/1
  Bus Selector2/1 -> Bus Creator/1  "<ESC_LatAcc>"
  Bus Selector2/2 -> Bus Creator/2  "<ESC_LatAcc_Valid>"
  Bus Selector2/3 -> Bus Creator/3  "<ESC_YawRate>"
  Bus Selector2/4 -> Bus Creator/4  "<ESC_YawRate_Valid>"
  Bus Selector2/5 -> Bus Creator/5  "<ESC_UnYawRate>"
  Bus Selector2/6 -> Bus Creator/6  "<ESC_VehSpd>"
  Bus Selector2/7 -> Bus Creator/7  "<ESC_LonAcc>"
  Bus Selector2/8 -> Bus Creator/8  "<ESC_LonAcc_Valid>"
  Bus Selector2/9 -> Bus Creator/9  "<ESC_Brake_Press>"
  Bus Selector2/10 -> Bus Creator/10  "<ESC_VehSpd_Valid>"
  Bus Creator/1 -> bsVehMovInfoOut/1

== system D53_LKAS/LL/LLOn/LDW ==
  LDW_stLDWActvFlg : Inport
  LDW_bsInInfoSyn : Inport  Port=2
  LDW_bsLDWClb : Inport  Port=3
  states : EnablePort  StatesWhenEnabling=reset
      settings: AttributesFormatString=states = %<StatesWhenEnabling>
  Bus Selector : BusSelector  OutputSignals=bsLaneInfo.bsL0Info.L0_C1,bsLaneInfo.bsR0Info.R0_C1
  Bus Selector1 : BusSelector  OutputSignals=LL_LDWS_SUPPRESS_HEADING
  Heading Angle Detection (HdAgDet) : Subsystem  Description=|
      | Block Name: Heading Angle Detection
      | Ab.: HdAgDet
      | No.: 1.3.1.0
      | Rev: 0.0.1
      | Update Date: 19-3-26
  LDWWarnInfo : MATLAB Function  TreatAsAtomicUnit=on
  LDW_Flag : Outport  OutputWhenDisabled=reset  InitialOutput=0
  wires:
  LDWWarnInfo/1(LDWWarnInfo) -> LDW_Flag/1
  Heading Angle Detection (HdAgDet)/1(HdAgDet_stHdAgDetFlg) -> LDWWarnInfo/2(LDW_stHdAgDetFlg)
  Bus Selector1/1 -> Heading Angle Detection (HdAgDet)/4(HdAgDet_phiHdAgThres_C)  "<LL_LDWS_SUPPRESS_HEADING>"
  LDW_bsLDWClb/1 -> Bus Selector1/1
  Bus Selector/2 -> Heading Angle Detection (HdAgDet)/3(HdAgDet_phiHdAgRgt)  "<R0_C1>"
  Bus Selector/1 -> Heading Angle Detection (HdAgDet)/2(HdAgDet_phiHdAgLft)  "<L0_C1>"
  LDW_stLDWActvFlg/1 -> LDWWarnInfo/1(LDW_stLDWActvFlg), Heading Angle Detection (HdAgDet)/1(HdAgDet_stLDWActvFlg)
  LDW_bsInInfoSyn/1 -> Bus Selector/1

== system D53_LKAS/LL/LLOn/LKA ==
  LKA_bsInInfoSyn : Inport
  LKA_bsLKAInPInfo : Inport  Port=2
  LKA_bsLKAClb : Inport  Port=3
  LKA_bsConstantClb : Inport  Port=4
  states = reset : EnablePort  StatesWhenEnabling=reset  ShowOutputPort=on
  Bus Selector : BusSelector  OutputSignals=LKA_SampleTime
  Cast To Single : DataTypeConversion  OutDataTypeStr=uint8
  Driver Torque Addition (DTA) : Subsystem
  LKA Exit Processing (LKAExPrcs) : Subsystem  Description=|
      | Block Name: LKA Exit Processing 
      | Ab.: LKAExPrcs
      | No.: 1.2.2.0
      | Rev: 0.0.1
      | Update Date: 19-5-13
  "LKA Motion Planning (LKAMP) " : Subsystem  Description=|
      | Block Name: LKA Motion Planning
      | Ab.: LKAMP
      | No.: 1.2.3.0
      | Rev: 0.0.1
      | Update Date: 19-5-13
  LKA SWA Limit (LKASWALim) : Subsystem  Description=|
      | Block Name: LKA SWA Synthesis
      | Ab.: LKASWASyn
      | No.: 1.2.6.0
      | Rev: 0.0.1
      | Update Date: 19-5-13
  LKA_Mon : Subsystem
  Lane Following (LF) : Subsystem  Description=|
      | Block Name: Lane Following
      | Ab.: LF
      | No.: 02
      | Rev: 00.00.01
      | Update Date: 19-3-28
  Plan To LaneFollowing (PTLF) : Subsystem
  LKA_ExitFlg : Outport  OutputWhenDisabled=reset  InitialOutput=0
  LKA_phiSWACmd : Outport  Port=2  OutputWhenDisabled=reset  InitialOutput=0
  LKA_M : Outport  Port=3  OutputWhenDisabled=reset  InitialOutput=0
  LKAMon : Outport  Port=4  OutputWhenDisabled=reset  InitialOutput=0
  tag scope: ActFlg=global, ActFlg_Mon=global, Ff=global, LKA_ConstantClb=global, LKA_SampleTime=global, PT1=global
  wires:
  LKA_Mon/1(LKAMon) -> LKAMon/1
  "LKA Motion Planning (LKAMP) "/2(LKAMP_tiT1) -> [PT1]  "PlanT1"
  "LKA Motion Planning (LKAMP) "/3(LKAMP_tiT2) -> ?  "PlanT2"
  "LKA Motion Planning (LKAMP) "/1(LKAMP_phiSWACmd) -> [Plan]  "PlanSWACmd"
  Lane Following (LF)/4(LF_phiDiffSWACmd) -> [D]
  Lane Following (LF)/2(LF_phiPropSWACmd) -> [P]
  Lane Following (LF)/1(LF_phiFfLFSWACmd) -> [Ff]
  Lane Following (LF)/3(LF_phiIntegSWACmd) -> [I]
  Driver Torque Addition (DTA)/2(DTA_M) -> LKA_M/1
  [LKAInPInfo] -> Lane Following (LF)/2(LF_bsLKAInPInfo)
  [Ff] -> LKA SWA Limit (LKASWALim)/2(LKASWALim_Ff)
  [LKA_bsInInfoSyn] -> Lane Following (LF)/1(LF_bsInInfoSyn)
  [LKA_bsInInfoSyn] -> Driver Torque Addition (DTA)/1(DTA_bsInInfoSyn)
  [LKA_bsInInfoSyn] -> "LKA Motion Planning (LKAMP) "/1(LKAMP_bsInInfoSyn)
  [LKA_bsInInfoSyn] -> LKA Exit Processing (LKAExPrcs)/1(LKAExPrcs_bsInInfoSyn)
  LKA_bsInInfoSyn/1 -> [LKA_bsInInfoSyn]
  [LKA_bsLKAClb] -> LKA SWA Limit (LKASWALim)/4(LKASWALim_bsLKAClb)
  [LKA_bsLKAClb] -> Lane Following (LF)/3(LF_bsLFClb)
  [LKA_bsLKAClb] -> Driver Torque Addition (DTA)/2(DTA_bsLFClb)
  [LKA_bsLKAClb] -> "LKA Motion Planning (LKAMP) "/4(LKAMP_bsLKAClb)
  [LKA_bsLKAClb] -> LKA Exit Processing (LKAExPrcs)/3(LKAExPrcs_bsLKAClb)
  [LKAInPInfo] -> LKA SWA Limit (LKASWALim)/3(LKASWALim_bsLKAInPInfo)
  LKA_bsLKAClb/1 -> [LKA_bsLKAClb]
  [LKAInPInfo] -> Plan To LaneFollowing (PTLF)/1(InP)
  [LKAInPInfo] -> LKA Exit Processing (LKAExPrcs)/2(LKAExPrcs_bsLKAInPInfo)
  [LKAInPInfo] -> "LKA Motion Planning (LKAMP) "/3(LKAMP_bsLKAInPInfo)
  LKA_bsLKAInPInfo/1 -> [LKAInPInfo]
  [LKA_ConstantClb] -> Lane Following (LF)/4(LF_bsConstantClb)
  [LKA_ConstantClb] -> "LKA Motion Planning (LKAMP) "/5(LLClb_bsConstantClb)
  [ActFlg] -> "LKA Motion Planning (LKAMP) "/2(LKAMP_stLKAActvFlg)
  [PT1] -> LKA Exit Processing (LKAExPrcs)/4(LKAExPrcs_PlanT1)
  [PT1] -> Plan To LaneFollowing (PTLF)/3(T1)
  [Plan] -> Plan To LaneFollowing (PTLF)/2(Plan)
  [DT] -> Plan To LaneFollowing (PTLF)/4(DrvTrq)
  Driver Torque Addition (DTA)/1(DTA_phiDTASWACmd) -> [DT]  "DT"
  [D] -> Plan To LaneFollowing (PTLF)/8(D)
  [I] -> Plan To LaneFollowing (PTLF)/7(I)
  [P] -> Plan To LaneFollowing (PTLF)/6(P)
  [Ff] -> Plan To LaneFollowing (PTLF)/5(Ff)
  LKA Exit Processing (LKAExPrcs)/1(LKAExPrcs_stExFlg) -> LKA_ExitFlg/1
  LKA SWA Limit (LKASWALim)/1(LKASWALim_phiSWACmd) -> LKA_phiSWACmd/1  "phiSWACmd"
  states = reset/1 -> Cast To Single/1
  Plan To LaneFollowing (PTLF)/1(SWACmd) -> LKA SWA Limit (LKASWALim)/1(LKASWALim_phiTFCSWACmd)  "PTLFSWACmd"
  Cast To Single/1 -> [ActFlg_Mon], [ActFlg]  "ActFlg"
  LKA_bsConstantClb/1 -> [LKA_ConstantClb], Bus Selector/1
  Bus Selector/1 -> [LKA_SampleTime]  "<LKA_SampleTime>"

== system D53_LKAS/LL/LLOn/LKA Input Processing (LKAInP) ==
  LKAInP_stLKAActvFlg : Inport
  LKAInP_bsInInfoSyn : Inport  Port=2
  LKAInP_bsLKAClb : Inport  Port=3
  Bus Creator : BusCreator  Inputs=6
  Bus Creator1 : BusCreator  Inputs=3
  Delay : Delay  DelayLength=1
  Lane Width Calculation (LW) : Subsystem
  Predicted Deviation Calculation (PrDvt) : Subsystem
  Predicted Heading Angle Calculation (PrHdAg) : Subsystem
  Previewed Curvature (PrCrvt) : Subsystem
  Steering Wheel Position Calculation (SWAPosCal) : Subsystem
  TTLC Calculation (TTLCCalc) : Subsystem  Description=|
      | Block Name: TTLC Calculation
      | Ab.: TTLCCalc
      | No.: 1.1.1.1
      | Rev: 0.0.1
      | Update Date: 19-3-26
  Under The Limit (UndrLim) : Subsystem
  LKAInP_bsLKAInPInfo : Outport
  wires:
  TTLC Calculation (TTLCCalc)/1(TTLCCalc_bsTTLCInfo) -> Predicted Heading Angle Calculation (PrHdAg)/1(PrHdAg_bsTTLCInfo), Bus Creator/2  "TTLC_bsTTLCInfo"
  Lane Width Calculation (LW)/1(LW_LaneWidth) -> Bus Creator/1  "LW_LaneWidth"
  Steering Wheel Position Calculation (SWAPosCal)/1(SWAPosCal) -> Bus Creator/6  "LKAInP_phiSWAPos"
  LKAInP_stLKAActvFlg/1 -> Delay/1
  Under The Limit (UndrLim)/2(UndrLim_dphiSWARMax) -> Bus Creator/5  "UndrLim_dphiSWARMax"
  Under The Limit (UndrLim)/1(UndrLim_phiSWAMax) -> Bus Creator/4  "UndrLim_phiSWAMax"
  Bus Creator1/1 -> Bus Creator/3  "Pr_bsPrInfo"
  Previewed Curvature (PrCrvt)/1(PrvwCrvt_bsPrvwCrvtInfo) -> Bus Creator1/3, TTLC Calculation (TTLCCalc)/3(bsPrvwCrvtInfo)  "bsPrCrvtInfo"
  Predicted Deviation Calculation (PrDvt)/1(PrdcDvt_bsPrdcDvtInfo) -> Bus Creator1/1, TTLC Calculation (TTLCCalc)/2(bsPrDvtInfo)  "bsPrDvtInfo"
  Predicted Heading Angle Calculation (PrHdAg)/1(PrHdAg_bsPrHdAgInfo) -> Bus Creator1/2, Predicted Deviation Calculation (PrDvt)/3(PrdcDvt_bsPrdcHdAgInfo)  "bsPrHdAgInfo"
  LKAInP_bsLKAClb/1 -> Predicted Deviation Calculation (PrDvt)/4(PrdcDvt_bsLKAClb), Predicted Heading Angle Calculation (PrHdAg)/4(PrHdAg_bsLKAClb), Previewed Curvature (PrCrvt)/3(PrvwCrvt_tiCrvtPrvwT_C), Under The Limit (UndrLim)/2(UndrLim_bsUndrLimClb)
  Bus Creator/1 -> LKAInP_bsLKAInPInfo/1
  LKAInP_bsInInfoSyn/1 -> Lane Width Calculation (LW)/1(LW_bsInInfoSyn), TTLC Calculation (TTLCCalc)/1(bsInfo), Predicted Deviation Calculation (PrDvt)/2(PrdcDvt_bsInInfoSyn), Predicted Heading Angle Calculation (PrHdAg)/3(PrHdAg_bsInInfoSyn), Previewed Curvature (PrCrvt)/2(PrvwCrvt_bsInInfoSyn), Under The Limit (UndrLim)/1(UndrLim_bsInInfoSyn), Steering Wheel Position Calculation (SWAPosCal)/1(SWAPosCal_bsInInfoSyn)
  Delay/1 -> Predicted Deviation Calculation (PrDvt)/1(PrdcDvt_stLKAActvFlg), Predicted Heading Angle Calculation (PrHdAg)/2(PrdcHdAg_stLKAActvFlg), Previewed Curvature (PrCrvt)/1(PrvwCrvt_stLKAActvFlg)

== system D53_LKAS/LL/LLOn/LL State Determination (LLStateDet) ==
  LLStateDet_stDACMode : Inport
  LLStateDet_bsInInfoSyn : Inport  Port=2
  LLStateDet_bsLKAInPInfo : Inport  Port=3
  LLStateDet_bsLLSMConClb : Inport  Port=4
  LLStateDet_stExitFlg : Inport  Port=5
  LLStateDet_SignalFault : Inport  Port=6
  Bus Creator : BusCreator  Inputs=3
  Delay : Delay  DelayLength=1
  Delay1 : Delay  DelayLength=1
  LDW_State_Machine : Stateflow chart  Description=|  TreatAsAtomicUnit=on
      | Block Name: LDW State Machine
      | Ab.: LDWSM
      | No.: 1.1.2.0
      | Rev: 0.0.1
      | Update Date: 19-3-26
      settings: RTWSystemCode=Nonreusable function
  LKA_State_Machine : Stateflow chart  Description=|  TreatAsAtomicUnit=on
      | Block Name: LKA State Machine
      | Ab.: LKASM
      | No.: 1.1.3.0
      | Rev: 0.0.1
      | Update Date: 19-3-26
      settings: RTWSystemCode=Nonreusable function
  LL State Machine Conditions (LLSMCon) : Subsystem
  LLStateDet_bsLLState : Outport
  LLStateDet_stLDWActvFlg : Outport  Port=2
  LLStateDet_stLKAActvFlg : Outport  Port=3
  tag scope: LDW_State_Mon=global, LKA_State_Mon=global
  wires:
  LLStateDet_SignalFault/1 -> LL State Machine Conditions (LLSMCon)/7(LLSMCon_bsSignalFault)
  Delay/1 -> LL State Machine Conditions (LLSMCon)/6(LLSMCon_stExitFlg)
  LLStateDet_bsLLSMConClb/1 -> LL State Machine Conditions (LLSMCon)/4(LLSMCon_bsLLSMConClb)
  LLStateDet_stExitFlg/1 -> Delay/1
  LLStateDet_stDACMode/1 -> LL State Machine Conditions (LLSMCon)/1(LLSMCon_stDACModeIn)
  LLStateDet_bsLKAInPInfo/1 -> LL State Machine Conditions (LLSMCon)/3(LLSMCon_bsLKAInPInfo)
  LLStateDet_bsInInfoSyn/1 -> LL State Machine Conditions (LLSMCon)/2(LLSMCon_bsInInfoSyn)
  LL State Machine Conditions (LLSMCon)/11(LLSMCon_stLKAFaultCSyn) -> LKA_State_Machine/6(LKASM_stFaultCSyn)
  LL State Machine Conditions (LLSMCon)/10(LLSMCon_stLKADeactvCSyn) -> LKA_State_Machine/5(LKASM_stDeactvCSyn)
  LL State Machine Conditions (LLSMCon)/9(LLSMCon_stLKAActvCSyn) -> LKA_State_Machine/4(LKASM_stActvCSyn)
  LL State Machine Conditions (LLSMCon)/8(LLSMCon_stLKADisblCSyn) -> LKA_State_Machine/3(LKASM_stDisblCSyn)
  LL State Machine Conditions (LLSMCon)/7(LLSMCon_stLKAEnaCSyn) -> LKA_State_Machine/2(LKASM_stEnaCSyn)
  LL State Machine Conditions (LLSMCon)/6(LLSMCon_stLDWFaultCSyn) -> LDW_State_Machine/6(LDWSM_stFaultCSyn)
  LDW_State_Machine/2(LDWSM_stLDWState) -> Bus Creator/1, [LDW_State_Mon]  "LDW_State"
  LKA_State_Machine/2(LKASM_stLKAState) -> Bus Creator/3, [LKA_State_Mon]  "LKA_State"
  Bus Creator/1 -> LLStateDet_bsLLState/1, Delay1/1  "LLState"
  Delay1/1 -> LL State Machine Conditions (LLSMCon)/5(LLSMCon_bsLLState)
  LKA_State_Machine/1(LKASM_stLKAActvFlg) -> LLStateDet_stLKAActvFlg/1
  LDW_State_Machine/1(LDWSM_stLDWActvFlg) -> LLStateDet_stLDWActvFlg/1
  LL State Machine Conditions (LLSMCon)/1(LLSMCon_stDACMode) -> LDW_State_Machine/1(LDWSM_stLMCMode), Bus Creator/2, LKA_State_Machine/1(LKASM_stLMCMode)  "DACMode"
  LL State Machine Conditions (LLSMCon)/5(LLSMCon_stLDWDeactvCSyn) -> LDW_State_Machine/5(LDWSM_stDeactvCSyn)
  LL State Machine Conditions (LLSMCon)/4(LLSMCon_stLDWActvCSyn) -> LDW_State_Machine/4(LDWSM_stActvCSyn)
  LL State Machine Conditions (LLSMCon)/3(LLSMCon_stLDWDisblCSyn) -> LDW_State_Machine/3(LDWSM_stDisblCSyn)
  LL State Machine Conditions (LLSMCon)/2(LLSMCon_stLDWEnaCSyn) -> LDW_State_Machine/2(LDWSM_stEnaCSyn)

== system D53_LKAS/LL/LLOn/LL_Mon ==
  LKAMon : Inport
  Bus : BusCreator  Inputs=3
  BusInP : BusCreator  Inputs=2
  BusState : BusCreator  Inputs=2
  LLMon : Outport
  wires:
  BusState/1 -> [StateMon]  "StateMon"
  BusInP/1 -> [InPMon]  "InPMon"
  [LKA_State_Mon] -> BusState/2  "LKA_State_Mon"
  [LDW_State_Mon] -> BusState/1  "LDW_State_Mon"
  [RGTTTLC_Mon] -> BusInP/2  "RGTTTLC_Mon"
  [LFTTTLC_Mon] -> BusInP/1  "LFTTTLC_Mon"
  Bus/1 -> LLMon/1  "LLMon"
  LKAMon/1 -> Bus/3
  [StateMon] -> Bus/2
  [InPMon] -> Bus/1

== system D53_LKAS/LLClb/LLSMConClb/ICv to v ==
  In1 : Inport
  Add : Sum  Inputs=+-
  Constant : Constant  Value=2.5  OutDataTypeStr=single
  Gain : Gain  Gain=1/1.02
  Out1 : Outport
  wires:
  Gain/1 -> Out1/1
  Constant/1 -> Add/2
  Add/1 -> Gain/1
  In1/1 -> Add/1

== system D53_LKAS/LLClb/LLSMConClb/ICv to v1 ==
  In1 : Inport
  Add : Sum  Inputs=+-
  Constant : Constant  Value=2.5  OutDataTypeStr=single
  Gain : Gain  Gain=1/1.02
  Out1 : Outport
  wires:
  In1/1 -> Add/1
  Add/1 -> Gain/1
  Constant/1 -> Add/2
  Gain/1 -> Out1/1

== system D53_LKAS/LLClb/LLSMConClb/ICv to v2 ==
  In1 : Inport
  Add : Sum  Inputs=+-
  Constant : Constant  Value=2.5  OutDataTypeStr=single
  Gain : Gain  Gain=1/1.02
  Out1 : Outport
  wires:
  Gain/1 -> Out1/1
  Constant/1 -> Add/2
  Add/1 -> Gain/1
  In1/1 -> Add/1

== system D53_LKAS/LLClb/LLSMConClb/ICv to v3 ==
  In1 : Inport
  Add : Sum  Inputs=+-
  Constant : Constant  Value=2.5  OutDataTypeStr=single
  Gain : Gain  Gain=1/1.02
  Out1 : Outport
  wires:
  In1/1 -> Add/1
  Add/1 -> Gain/1
  Constant/1 -> Add/2
  Gain/1 -> Out1/1

== system D53_LKAS/LLClb/LLSMConClb/ICv to v4 ==
  In1 : Inport
  Add : Sum  Inputs=+-
  Constant : Constant  Value=2.5  OutDataTypeStr=single
  Gain : Gain  Gain=1/1.02
  Out1 : Outport
  wires:
  Gain/1 -> Out1/1
  Constant/1 -> Add/2
  Add/1 -> Gain/1
  In1/1 -> Add/1

== system D53_LKAS/LLClb/LLSMConClb/ICv to v5 ==
  In1 : Inport
  Add : Sum  Inputs=+-
  Constant : Constant  Value=2.5  OutDataTypeStr=single
  Gain : Gain  Gain=1/1.02
  Out1 : Outport
  wires:
  In1/1 -> Add/1
  Add/1 -> Gain/1
  Constant/1 -> Add/2
  Gain/1 -> Out1/1

== system D53_LKAS/Clb/Calibration1/Subsystem2/If Action Subsystem ==
  In1 : Inport
  Action Port : ActionPort  ActionType=then
  Out1 : Outport
  wires:
  In1/1 -> Out1/1

== system D53_LKAS/Clb/Calibration1/Subsystem2/If Action Subsystem1 ==
  In1 : Inport
  Action Port : ActionPort  ActionType=elseif
  Out1 : Outport
  wires:
  In1/1 -> Out1/1

== system D53_LKAS/Clb/Calibration1/Subsystem2/If Action Subsystem2 ==
  In1 : Inport
  Action Port : ActionPort  ActionType=elseif
  Out1 : Outport
  wires:
  In1/1 -> Out1/1

== system D53_LKAS/Clb/Calibration1/Subsystem2/If Action Subsystem3 ==
  In1 : Inport
  Action Port : ActionPort  ActionType=elseif
  Out1 : Outport
  wires:
  In1/1 -> Out1/1

== system D53_LKAS/Clb/Calibration1/Subsystem2/If Action Subsystem4 ==
  In1 : Inport
  Action Port : ActionPort  ActionType=elseif
  Out1 : Outport
  wires:
  In1/1 -> Out1/1

== system D53_LKAS/Clb/Calibration1/Subsystem2/If Action Subsystem5 ==
  In1 : Inport
  Action Port : ActionPort  ActionType=elseif
  Out1 : Outport
  wires:
  In1/1 -> Out1/1

== system D53_LKAS/Clb/Calibration1/Subsystem2/If Action Subsystem6 ==
  In1 : Inport
  Action Port : ActionPort  ActionType=elseif
  Out1 : Outport
  wires:
  In1/1 -> Out1/1

== system D53_LKAS/Clb/Calibration1/Subsystem2/If Action Subsystem7 ==
  In1 : Inport
  Action Port : ActionPort  ActionType=elseif
  Out1 : Outport
  wires:
  In1/1 -> Out1/1

== system D53_LKAS/Clb/Calibration1/Subsystem2/If Action Subsystem8 ==
  In1 : Inport
  Action Port : ActionPort  ActionType=elseif
  Out1 : Outport
  wires:
  In1/1 -> Out1/1

== system D53_LKAS/Clb/Calibration1/Subsystem2/If Action Subsystem9 ==
  In1 : Inport
  Action Port : ActionPort  ActionType=elseif
  Out1 : Outport
  wires:
  In1/1 -> Out1/1

== system D53_LKAS/Clb/Calibration2/Subsystem2/If Action Subsystem ==
  In1 : Inport
  Action Port : ActionPort  ActionType=then
  Out1 : Outport
  wires:
  In1/1 -> Out1/1

== system D53_LKAS/Clb/Calibration2/Subsystem2/If Action Subsystem1 ==
  In1 : Inport
  Action Port : ActionPort  ActionType=elseif
  Out1 : Outport
  wires:
  In1/1 -> Out1/1

== system D53_LKAS/Clb/Calibration2/Subsystem2/If Action Subsystem2 ==
  In1 : Inport
  Action Port : ActionPort  ActionType=elseif
  Out1 : Outport
  wires:
  In1/1 -> Out1/1
